simulink model "transor"  (R2013a)
settings: Solver=ode45  StartTime=0.0  StopTime=10.0  RelTol=1e-3
libraries: powerlib x5
settings Model: Creator=Christian  LastModifiedBy=Christian

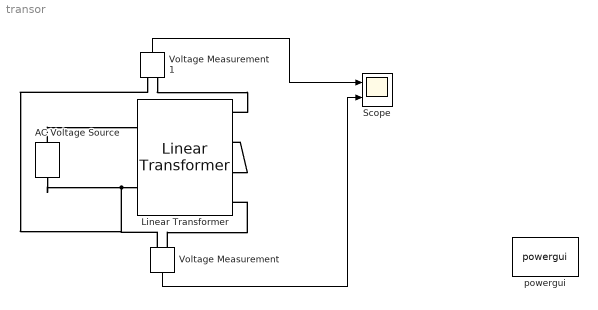
== system transor ==
  AC Voltage Source : powerlib/Electrical Sources/AC Voltage Source  Amplitude=100  Phase=0  Frequency=60  SampleTime=0  Measurements=Voltage
  Linear Transformer : powerlib/Elements/Linear Transformer  LConnTagsString=a|b  RConnTagsString=A|B|C|D  UNITS=pu  NominalPower=[ 250e6 60 ]  winding1="[ 735e3  0.002  0.08 ]"  winding2="[ 315e3  0.002  0.08 ]"  ThreeWindings=on  winding3=[ 315e3 0.002 0.08 ]  RmLm=[ 500 500 ]  Measurements=None  DataType=off
  Scope : Scope  NumInputPorts=2
      settings: TimeRange=10  YMin=-5~-5  YMax=5~5
  Voltage Measurement : powerlib/Measurements/Voltage Measurement  PhasorSimulation=off  OutputType=Complex  PSBequivalent=0
  Voltage Measurement1 : powerlib/Measurements/Voltage Measurement  PhasorSimulation=off  OutputType=Complex  PSBequivalent=0
  powergui : powerlib/powergui  Priority=1  SimulationMode=Continuous  SolverType=Tustin  SampleTime=50e-6  frequency=60  SPID=off  DisableSnubberDevices=off  DisableRonSwitches=off  DisableVfSwitches=off  SwTol=0  Interpol=off  DisplayEquations=off  frequencyindice=60  Pbase=100e6  ErrMax=1e-4  Iterations=50  UnitsV=kV  UnitsW=MW  FunctionMessages=off  echomessages=off  HookPort=off  EnableUseOfTLC=off  x0status=blocks  RestoreLinks=warning  ResistiveCurrentMeasurement=off  Frange=[0:2:500]  Ylog=off  Xlog=on  ShowGrid=off  save=off  variable=ZData  ZoomFFT=off  StartTime=0.0  cycles=1  DisplayStyle=1  fundamental=60  FreqAxis=off  MaxFrequency=1000  frequencyindicesteady=1  RmsSteady=1  display=off  Ts=0  methode=off
  wires:
  Voltage Measurement1/1 -> Scope/1
  Voltage Measurement/1 -> Scope/2
  connections:
  Linear Transformer/RConn3 -- Linear Transformer/RConn2
  AC Voltage Source/RConn1 -- Linear Transformer/LConn1
  AC Voltage Source/LConn1 -- Voltage Measurement1/LConn1 -- Voltage Measurement/LConn1 -- Linear Transformer/LConn2
  Voltage Measurement1/LConn2 -- Linear Transformer/RConn1
  Voltage Measurement/LConn2 -- Linear Transformer/RConn4
